simulink model "prob7"  (R2020b)
settings: Solver=VariableStepAuto  StartTime=0.0  StopTime=10.0  RelTol=1e-3
settings Model: OrderedModelArguments=off  Creator=Admin  LastModifiedBy=Admin

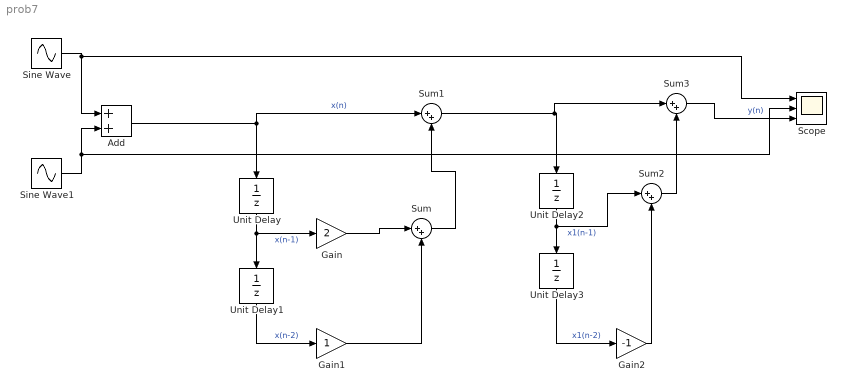
== system prob7 ==
  Add : Sum
  Gain : Gain  Gain=2
  Gain1 : Gain
  Gain2 : Gain  Gain=-1
  Scope : Scope  NumInputPorts=3
  Sine Wave : Sin  SampleTime=0
  Sine Wave1 : Sin  Frequency=50  SampleTime=0
  Sum{,1..3} (4 alike) : Sum  Inputs=|++
  Unit Delay{,1..3} (4 alike) : UnitDelay  SampleTime=-1  HasFrameUpgradeWarning=on
  wires:
  Add/1 -> Sum1/1, Unit Delay/1  "x(n)"
  Unit Delay/1 -> Gain/1, Unit Delay1/1  "x(n-1)"
  Unit Delay1/1 -> Gain1/1  "x(n-2)"
  Gain/1 -> Sum/1
  Gain1/1 -> Sum/2
  Sum/1 -> Sum1/2
  Sum1/1 -> Unit Delay2/1, Sum3/1
  Unit Delay2/1 -> Sum2/1, Unit Delay3/1  "x1(n-1)"
  Unit Delay3/1 -> Gain2/1  "x1(n-2)"
  Gain2/1 -> Sum2/2
  Sum2/1 -> Sum3/2
  Sine Wave/1 -> Scope/1, Add/1
  Sine Wave1/1 -> Scope/2, Add/2
  Sum3/1 -> Scope/3  "y(n)"
